simulink model "SF049A_LoaMgr"  (R2013b)
settings: Solver=FixedStepDiscrete  SolverMode=SingleTasking  StartTime=0.0  StopTime=1  FixedStep=0.002  RelTol=1e-3
values from neighbouring files (symbols this model uses):
  CURRMEASLOAMTGTNMASK_CNT_U08 = DataDict.Constant    [SF049A_LoaMgr_DataDict.m]
  IVTRLOAMTGTNMASK_CNT_U08 = DataDict.Constant    [SF049A_LoaMgr_DataDict.m]
  LOAMAXSLEW_ULSPERSEC_F32 = DataDict.Constant    [SF049A_LoaMgr_DataDict.m]
  LoaMgrCurrIvtrMtgtnRate = DataDict.Calibration    [SF049A_LoaMgr_DataDict.m]
  LoaMgrCurrIvtrMtgtnSca = DataDict.Calibration    [SF049A_LoaMgr_DataDict.m]
  LoaMgrCurrIvtrMtgtnScaZeroEna = DataDict.Calibration    [SF049A_LoaMgr_DataDict.m]
  LoaMgrCurrMeasIdptSig0Resp = DataDict.Calibration    [SF049A_LoaMgr_DataDict.m]
  LoaMgrCurrMeasIdptSig1Resp = DataDict.Calibration    [SF049A_LoaMgr_DataDict.m]
  LoaMgrCurrMeasIdptSig2Resp = DataDict.Calibration    [SF049A_LoaMgr_DataDict.m]
  LoaMgrCurrMeasIdptSigFltThd = DataDict.Calibration    [SF049A_LoaMgr_DataDict.m]
  LoaMgrCurrMeasMtgtnRate = DataDict.Calibration    [SF049A_LoaMgr_DataDict.m]
  LoaMgrCurrMeasMtgtnSca = DataDict.Calibration    [SF049A_LoaMgr_DataDict.m]
  LoaMgrCurrMeasMtgtnScaZeroEna = DataDict.Calibration    [SF049A_LoaMgr_DataDict.m]
  LoaMgrFadeOutStRate = DataDict.Calibration    [SF049A_LoaMgr_DataDict.m]
  LoaMgrHwTqIdptSig0NoTqLoaResp = DataDict.Calibration    [SF049A_LoaMgr_DataDict.m]
  LoaMgrHwTqIdptSig1NoTqLoaResp = DataDict.Calibration    [SF049A_LoaMgr_DataDict.m]
  LoaMgrHwTqIdptSig2Resp = DataDict.Calibration    [SF049A_LoaMgr_DataDict.m]
  LoaMgrHwTqIdptSig4Resp = DataDict.Calibration    [SF049A_LoaMgr_DataDict.m]
  LoaMgrHwTqIdptSigFltThd = DataDict.Calibration    [SF049A_LoaMgr_DataDict.m]
  LoaMgrHwTqLoaAvlResp = DataDict.Calibration    [SF049A_LoaMgr_DataDict.m]
  LoaMgrIvtrIdptSig0Resp = DataDict.Calibration    [SF049A_LoaMgr_DataDict.m]
  LoaMgrIvtrIdptSig1Resp = DataDict.Calibration    [SF049A_LoaMgr_DataDict.m]
  LoaMgrIvtrIdptSig2Resp = DataDict.Calibration    [SF049A_LoaMgr_DataDict.m]
  LoaMgrIvtrIdptSigFltThd = DataDict.Calibration    [SF049A_LoaMgr_DataDict.m]
  LoaMgrIvtrMtgtnRate = DataDict.Calibration    [SF049A_LoaMgr_DataDict.m]
  LoaMgrIvtrMtgtnSca = DataDict.Calibration    [SF049A_LoaMgr_DataDict.m]
  LoaMgrIvtrMtgtnScaZeroEna = DataDict.Calibration    [SF049A_LoaMgr_DataDict.m]
  LoaMgrLimdStRate = DataDict.Calibration    [SF049A_LoaMgr_DataDict.m]
  LoaMgrLimdStSca = DataDict.Calibration    [SF049A_LoaMgr_DataDict.m]
  LoaMgrMotAgAvlSnsrlsResp = DataDict.Calibration    [SF049A_LoaMgr_DataDict.m]
  LoaMgrMotAgIdptSig0NoSnsrlsResp = DataDict.Calibration    [SF049A_LoaMgr_DataDict.m]
  LoaMgrMotAgIdptSig1NoSnsrlsResp = DataDict.Calibration    [SF049A_LoaMgr_DataDict.m]
  LoaMgrMotAgIdptSig2Resp = DataDict.Calibration    [SF049A_LoaMgr_DataDict.m]
  LoaMgrMotAgIdptSig3Resp = DataDict.Calibration    [SF049A_LoaMgr_DataDict.m]
  LoaMgrMotAgIdptSigFltThd = DataDict.Calibration    [SF049A_LoaMgr_DataDict.m]
  LoaMgrMotAgMtgtnRate = DataDict.Calibration    [SF049A_LoaMgr_DataDict.m]
  LoaMgrMotAgMtgtnSca = DataDict.Calibration    [SF049A_LoaMgr_DataDict.m]
  LoaMgrMotAgMtgtnScaZeroEna = DataDict.Calibration    [SF049A_LoaMgr_DataDict.m]
  LOASCAONE_ULS_F32 = DataDict.Constant    [SF049A_LoaMgr_DataDict.m]
  LOASCAZERO_ULS_F32 = DataDict.Constant    [SF049A_LoaMgr_DataDict.m]
  LOASTIMDTSHTDWN_CNT_U08 = DataDict.Constant    [SF049A_LoaMgr_DataDict.m]
  LOASTNORM_CNT_U08 = DataDict.Constant    [SF049A_LoaMgr_DataDict.m]
  LOASTSWMTGTN_CNT_U08 = DataDict.Constant    [SF049A_LoaMgr_DataDict.m]
  MAXCURRMEASIDPTSIGALLWD_CNT_U08 = DataDict.Constant    [SF049A_LoaMgr_DataDict.m]
  MAXHWTQIDPTSIGALLWD_CNT_U08 = DataDict.Constant    [SF049A_LoaMgr_DataDict.m]
  MAXIVTRIDPTSIGALLWD_CNT_U08 = DataDict.Constant    [SF049A_LoaMgr_DataDict.m]
  MAXMOTAGMECLIDPTSIGALLWD_CNT_U08 = DataDict.Constant    [SF049A_LoaMgr_DataDict.m]
  NODEBSTEP_CNT_U16 = DataDict.Constant    [SF049A_LoaMgr_DataDict.m]
undefined symbols (not defined in the file or in its folder): LoaSt1, NtcNr1, NtcSts1, SigQlfr1
libraries: simulink x43, NxtrMin x4, NxtrMax x4, NxtrLim x2
(part 7 of 8)

== system SF049A_LoaMgr/LoaMgr/LoaMgrPer1/Request_Responses/MotAgResp/one ==
  MotAgAvlSnsrlsResp : Inport
  MotAgIdptSig1NoResp : Inport  Port=2
  MotAgAvlSnsrls : Inport  Port=3
  one : ActionPort  ActionType=case
  " " : Merge  RequirementInfo="{'linktype_rmi_doors' '0000bab3 (/E-STEER Core/SubSystem Specifications/Application Functions/SF049A Loss of Assist Manager)' '#SF049A_183' 'true' 'REQ:  SF049A_183' '' } %GIDa_4182a502_c274_4352_b30c_44918a836976"
  CopyRight2 : Subsystem  Description=|  mask(Copyright Information){none=on}
      | Copyright info block.                                               
      |                                                                     
      | Place copyright information at the top of every subsystem in design.
      mask prompts: none "No parameters"
      mask help: Place copyright information at the top of every subsystem in design.
      mask Display:
      | NxtrConf = 'Nexteer Confidential';
      | 
      | sys = bdroot; %handle for the current model ("system")
      | first = get_param(sys,'Created');
      | first = first(end-3:end);  %year is last four digits
      | 
      | last = get_param(sys,'LastModifiedDate');
      | if isempty(last)
      |     last = datestr(now,'yyyy');
      | else
      |     last = last(end-3:end);
      | end
      | 
      | if strcmp(first,last)
      |     fprintf('%s -- Copyright %s Nexteer',NxtrConf,first)
      | else
      |     fprintf('%s -- %s%s- %s Nexteer',NxtrConf,char(169),first,last)
      | end
  Ivtr1Inactv_IF : If  RequirementInfo="{'linktype_rmi_doors' '0000bab3 (/E-STEER Core/SubSystem Specifications/Application Functions/SF049A Loss of Assist Manager)' '#SF049A_183' 'true' 'REQ:  SF049A_183' '' } %GIDa_d9c4d673_0ab1_4232_be5c_95383af81f7c"  IfExpression=u1
  cal1 : Subsystem  RequirementInfo="{'linktype_rmi_doors' '0000bab3 (/E-STEER Core/SubSystem Specifications/Application Functions/SF049A Loss of Assist Manager)' '#SF049A_183' 'true' 'REQ:  SF049A_183' '' } %GIDa_64953195_8878_4b1c_98ab_73167e7d198e"  TreatAsAtomicUnit=on
      settings: RTWSystemCode=Inline
  cal2 : Subsystem  RequirementInfo="{'linktype_rmi_doors' '0000bab3 (/E-STEER Core/SubSystem Specifications/Application Functions/SF049A Loss of Assist Manager)' '#SF049A_183' 'true' 'REQ:  SF049A_183' '' } %GIDa_9b0a2cdc_50bc_461c_be5e_30bc8b3ac44b"  TreatAsAtomicUnit=on
      settings: RTWSystemCode=Inline
  MotAgResp : Outport
  wires:
  " "/1 -> MotAgResp/1
  MotAgIdptSig1NoResp/1 -> cal2/1(In1)
  MotAgAvlSnsrlsResp/1 -> cal1/1(In1)
  cal1/1(Out2) -> " "/1
  MotAgAvlSnsrls/1 -> Ivtr1Inactv_IF/1
  cal2/1(Out1) -> " "/2
  Ivtr1Inactv_IF/1 -> cal1/Action
  Ivtr1Inactv_IF/2 -> cal2/Action

== system SF049A_LoaMgr/LoaMgr/LoaMgrPer1/Set_Faults/NTC_Fault1/SetNtcSts ==
  NtcNr : Inport
  NtcStInfo : Inport  Port=2
  NtcSts : Inport  Port=3
  DebStep : Inport  Port=4
  CopyRight2 : Subsystem  Description=|  mask(Copyright Information){none=on}
      | Copyright info block.                                               
      |                                                                     
      | Place copyright information at the top of every subsystem in design.
      mask prompts: none "No parameters"
      mask help: Place copyright information at the top of every subsystem in design.
      mask Display:
      | NxtrConf = 'Nexteer Confidential';
      | 
      | sys = bdroot; %handle for the current model ("system")
      | first = get_param(sys,'Created');
      | first = first(end-3:end);  %year is last four digits
      | 
      | last = get_param(sys,'LastModifiedDate');
      | if isempty(last)
      |     last = datestr(now,'yyyy');
      | else
      |     last = last(end-3:end);
      | end
      | 
      | if strcmp(first,last)
      |     fprintf('%s -- Copyright %s Nexteer',NxtrConf,first)
      | else
      |     fprintf('%s -- %s%s- %s Nexteer',NxtrConf,char(169),first,last)
      | end
  Data Store Write1 : DataStoreWrite  DataStoreName=DebStep
  Data Store Write3 : DataStoreWrite  DataStoreName=Fault1_Status
  Terminator : Terminator
  Terminator1 : Terminator
  wires:
  NtcStInfo/1 -> Terminator1/1
  NtcNr/1 -> Terminator/1
  NtcSts/1 -> Data Store Write3/1
  DebStep/1 -> Data Store Write1/1

== system SF049A_LoaMgr/LoaMgr/LoaMgrPer1/Set_Faults/NTC_Fault2/SetNtcSts ==
  NtcNr : Inport
  NtcStInfo : Inport  Port=2
  NtcSts : Inport  Port=3
  DebStep : Inport  Port=4
  CopyRight2 : Subsystem  Description=|  mask(Copyright Information){none=on}
      | Copyright info block.                                               
      |                                                                     
      | Place copyright information at the top of every subsystem in design.
      mask prompts: none "No parameters"
      mask help: Place copyright information at the top of every subsystem in design.
      mask Display:
      | NxtrConf = 'Nexteer Confidential';
      | 
      | sys = bdroot; %handle for the current model ("system")
      | first = get_param(sys,'Created');
      | first = first(end-3:end);  %year is last four digits
      | 
      | last = get_param(sys,'LastModifiedDate');
      | if isempty(last)
      |     last = datestr(now,'yyyy');
      | else
      |     last = last(end-3:end);
      | end
      | 
      | if strcmp(first,last)
      |     fprintf('%s -- Copyright %s Nexteer',NxtrConf,first)
      | else
      |     fprintf('%s -- %s%s- %s Nexteer',NxtrConf,char(169),first,last)
      | end
  Data Store Write1 : DataStoreWrite  DataStoreName=DebStep
  Data Store Write3 : DataStoreWrite  DataStoreName=Fault2_Status
  Terminator : Terminator
  Terminator1 : Terminator
  wires:
  DebStep/1 -> Data Store Write1/1
  NtcSts/1 -> Data Store Write3/1
  NtcNr/1 -> Terminator/1
  NtcStInfo/1 -> Terminator1/1

== system SF049A_LoaMgr/LoaMgr/LoaMgrPer1/Set_Faults/NTC_Fault3/SetNtcSts ==
  NtcNr : Inport
  NtcStInfo : Inport  Port=2
  NtcSts : Inport  Port=3
  DebStep : Inport  Port=4
  CopyRight2 : Subsystem  Description=|  mask(Copyright Information){none=on}
      | Copyright info block.                                               
      |                                                                     
      | Place copyright information at the top of every subsystem in design.
      mask prompts: none "No parameters"
      mask help: Place copyright information at the top of every subsystem in design.
      mask Display:
      | NxtrConf = 'Nexteer Confidential';
      | 
      | sys = bdroot; %handle for the current model ("system")
      | first = get_param(sys,'Created');
      | first = first(end-3:end);  %year is last four digits
      | 
      | last = get_param(sys,'LastModifiedDate');
      | if isempty(last)
      |     last = datestr(now,'yyyy');
      | else
      |     last = last(end-3:end);
      | end
      | 
      | if strcmp(first,last)
      |     fprintf('%s -- Copyright %s Nexteer',NxtrConf,first)
      | else
      |     fprintf('%s -- %s%s- %s Nexteer',NxtrConf,char(169),first,last)
      | end
  Data Store Write1 : DataStoreWrite  DataStoreName=DebStep
  Data Store Write3 : DataStoreWrite  DataStoreName=Fault3_Status
  Terminator : Terminator
  Terminator1 : Terminator
  wires:
  DebStep/1 -> Data Store Write1/1
  NtcSts/1 -> Data Store Write3/1
  NtcNr/1 -> Terminator/1
  NtcStInfo/1 -> Terminator1/1

== system SF049A_LoaMgr/LoaMgr/LoaMgrPer1/Set_Faults/NTC_Fault4/SetNtcSts ==
  NtcNr : Inport
  NtcStInfo : Inport  Port=2
  NtcSts : Inport  Port=3
  DebStep : Inport  Port=4
  CopyRight2 : Subsystem  Description=|  mask(Copyright Information){none=on}
      | Copyright info block.                                               
      |                                                                     
      | Place copyright information at the top of every subsystem in design.
      mask prompts: none "No parameters"
      mask help: Place copyright information at the top of every subsystem in design.
      mask Display:
      | NxtrConf = 'Nexteer Confidential';
      | 
      | sys = bdroot; %handle for the current model ("system")
      | first = get_param(sys,'Created');
      | first = first(end-3:end);  %year is last four digits
      | 
      | last = get_param(sys,'LastModifiedDate');
      | if isempty(last)
      |     last = datestr(now,'yyyy');
      | else
      |     last = last(end-3:end);
      | end
      | 
      | if strcmp(first,last)
      |     fprintf('%s -- Copyright %s Nexteer',NxtrConf,first)
      | else
      |     fprintf('%s -- %s%s- %s Nexteer',NxtrConf,char(169),first,last)
      | end
  Data Store Write1 : DataStoreWrite  DataStoreName=DebStep
  Data Store Write3 : DataStoreWrite  DataStoreName=Fault4_Status
  Terminator : Terminator
  Terminator1 : Terminator
  wires:
  NtcStInfo/1 -> Terminator1/1
  NtcNr/1 -> Terminator/1
  NtcSts/1 -> Data Store Write3/1
  DebStep/1 -> Data Store Write1/1

== system SF049A_LoaMgr/LoaMgr/LoaMgrPer1/Set_Faults/NTC_Fault5/CopyRight2 ==

== system SF049A_LoaMgr/LoaMgr/LoaMgrPer1/Set_Faults/NTC_Fault6/CopyRight2 ==

== system SF049A_LoaMgr/LoaMgr/LoaMgrPer1/Arbitrate_Responses/CntSwBasdMtgtn/CntMtgtnReq/CopyRight2 ==

== system SF049A_LoaMgr/LoaMgr/LoaMgrPer1/Arbitrate_Responses/CntSwBasdMtgtn/CntMtgtnReq/HwTq_ELSE ==
  In1 : Inport
  Action Port : ActionPort  ActionType=else
  Out1 : Outport
  wires:
  In1/1 -> Out1/1

== system SF049A_LoaMgr/LoaMgr/LoaMgrPer1/Arbitrate_Responses/CntSwBasdMtgtn/CntMtgtnReq/HwTq_THEN ==
  In1 : Inport
  Action Port : ActionPort  ActionType=then
  Out1 : Outport
  wires:
  In1/1 -> Out1/1

== system SF049A_LoaMgr/LoaMgr/LoaMgrPer1/Arbitrate_Responses/CntSwBasdMtgtn/CntMtgtnReq/MotAg_ELSE ==
  In1 : Inport
  Action Port : ActionPort  ActionType=else
  Out1 : Outport
  wires:
  In1/1 -> Out1/1

== system SF049A_LoaMgr/LoaMgr/LoaMgrPer1/Arbitrate_Responses/CntSwBasdMtgtn/CntMtgtnReq/MotAg_THEN ==
  In1 : Inport
  Action Port : ActionPort  ActionType=then
  Out1 : Outport
  wires:
  In1/1 -> Out1/1

== system SF049A_LoaMgr/LoaMgr/LoaMgrPer1/Arbitrate_Responses/CntSwBasdMtgtn/CntMtgtnReq/VltgModReq_ELSE ==
  In1 : Inport
  Action Port : ActionPort  ActionType=else
  Out1 : Outport
  wires:
  In1/1 -> Out1/1

== system SF049A_LoaMgr/LoaMgr/LoaMgrPer1/Arbitrate_Responses/CntSwBasdMtgtn/CntMtgtnReq/VltgModReq_THEN ==
  In1 : Inport
  Action Port : ActionPort  ActionType=then
  Out1 : Outport
  wires:
  In1/1 -> Out1/1

== system SF049A_LoaMgr/LoaMgr/LoaMgrPer1/Arbitrate_Responses/CntSwBasdMtgtn/IllegalCombination/CopyRight2 ==

== system SF049A_LoaMgr/LoaMgr/LoaMgrPer1/Arbitrate_Responses/CntSwBasdMtgtn/OK_to_use/CopyRight2 ==

== system SF049A_LoaMgr/LoaMgr/LoaMgrPer1/Arbitrate_Responses/SelFinalResp/F1/CopyRight2 ==

== system SF049A_LoaMgr/LoaMgr/LoaMgrPer1/Arbitrate_Responses/SelFinalResp/F2/CopyRight2 ==

== system SF049A_LoaMgr/LoaMgr/LoaMgrPer1/Arbitrate_Responses/SelFinalResp/Fade_Out/CopyRight2 ==

== system SF049A_LoaMgr/LoaMgr/LoaMgrPer1/Arbitrate_Responses/SelFinalResp/Fade_Out1/CopyRight2 ==

== system SF049A_LoaMgr/LoaMgr/LoaMgrPer1/Arbitrate_Responses/SelFinalResp/Norm/CopyRight2 ==

== system SF049A_LoaMgr/LoaMgr/LoaMgrPer1/Arbitrate_Responses/SelFinalResp/Reduced/CopyRight2 ==

== system SF049A_LoaMgr/LoaMgr/LoaMgrPer1/Arbitrate_Responses/SelFinalResp/SwBasd_Mtgtn/CopyRight2 ==

== system SF049A_LoaMgr/LoaMgr/LoaMgrPer1/Assign_Scale/SwMtgtn/HwTqTrue/CopyRight2 ==

== system SF049A_LoaMgr/LoaMgr/LoaMgrPer1/Assign_Scale/SwMtgtn/MaskBooleans/CopyRight2 ==

== system SF049A_LoaMgr/LoaMgr/LoaMgrPer1/Assign_Scale/SwMtgtn/MaskBooleans/CurrMeas_ELSE ==
  In1 : Inport
  Action Port : ActionPort  ActionType=else
  Out1 : Outport
  wires:
  In1/1 -> Out1/1

== system SF049A_LoaMgr/LoaMgr/LoaMgrPer1/Assign_Scale/SwMtgtn/MaskBooleans/CurrMeas_THEN ==
  In1 : Inport
  Action Port : ActionPort  ActionType=then
  Out1 : Outport
  wires:
  In1/1 -> Out1/1

== system SF049A_LoaMgr/LoaMgr/LoaMgrPer1/Assign_Scale/SwMtgtn/MaskBooleans/Ivtr_ELSE ==
  In1 : Inport
  Action Port : ActionPort  ActionType=else
  Out1 : Outport
  wires:
  In1/1 -> Out1/1

== system SF049A_LoaMgr/LoaMgr/LoaMgrPer1/Assign_Scale/SwMtgtn/MaskBooleans/Ivtr_THEN ==
  In1 : Inport
  Action Port : ActionPort  ActionType=then
  Out1 : Outport
  wires:
  In1/1 -> Out1/1

== system SF049A_LoaMgr/LoaMgr/LoaMgrPer1/Assign_Scale/SwMtgtn/MotAgTrue/CopyRight2 ==

== system SF049A_LoaMgr/LoaMgr/LoaMgrPer1/Assign_Scale/SwMtgtn/MotAgTrue/PassThru1 ==
  In1 : Inport
  In2 : Inport  Port=2
  Action Port : ActionPort  ActionType=then
  Sca : Outport
  Rate : Outport  Port=2
  wires:
  In1/1 -> Sca/1
  In2/1 -> Rate/1

== system SF049A_LoaMgr/LoaMgr/LoaMgrPer1/Assign_Scale/SwMtgtn/MotAgTrue/PassThru2 ==
  In1 : Inport
  In2 : Inport  Port=2
  Action Port : ActionPort  ActionType=else
  Sca : Outport
  Rate : Outport  Port=2
  wires:
  In1/1 -> Sca/1
  In2/1 -> Rate/1

== system SF049A_LoaMgr/LoaMgr/LoaMgrPer1/Assign_Scale/SwMtgtn/OthersTrue/CopyRight2 ==

== system SF049A_LoaMgr/LoaMgr/LoaMgrPer1/Assign_Scale/SwMtgtn/OthersTrue/CurrIvtr ==
  NewValFlg : Inport  RequirementInfo="{'linktype_rmi_doors' '0000bab3 (/E-STEER Core/SubSystem Specifications/Application Functions/SF049A Loss of Assist Manager)' '#SF049A_107' 'true' 'REQ:  SF049A_107' '' } %GIDa_e92ac1af_0296_4258_8e06_232be688a8c1"
  Action Port : ActionPort  ActionType=case
  Constant1 : Constant  RequirementInfo="{'linktype_rmi_doors' '0000bab3 (/E-STEER Core/SubSystem Specifications/Application Functions/SF049A Loss of Assist Manager)' '#SF049A_104' 'true' 'REQ:  SF049A_104' '' ; 'linktype_rmi_doors' '0000bab3 (/E-STEER Core/SubSystem Specifications/Application Functions/SF049A Loss of Assist Manager)' '#SF049A_107' 'true' 'REQ:  SF049A_107' '' ; 'linktype_rmi_doors' '0000bab3 (/E-STEER Core/SubSystem Specifications/Application Functions/SF049A Loss of Assist Manager)' '#SF049A_108' 'true' 'REQ:  SF049A_108' '' } %GIDa_0a7f0acf_b35d_434a_8dc6_ba391d17eb63"  Value=LoaMgrCurrIvtrMtgtnRate
  Constant3 : Constant  RequirementInfo="{'linktype_rmi_doors' '0000bab3 (/E-STEER Core/SubSystem Specifications/Application Functions/SF049A Loss of Assist Manager)' '#SF049A_107' 'true' 'REQ:  SF049A_107' '' } %GIDa_4edd071c_4397_4e3b_a07a_efc9ca10b177"  Value=LOASCAZERO_ULS_F32
  Constant4 : Constant  RequirementInfo="{'linktype_rmi_doors' '0000bab3 (/E-STEER Core/SubSystem Specifications/Application Functions/SF049A Loss of Assist Manager)' '#SF049A_107' 'true' 'REQ:  SF049A_107' '' } %GIDa_e2b66e7c_9ee8_43b1_b96c_e0e22fd25a1e"  Value=LOAMAXSLEW_ULSPERSEC_F32
  Constant5 : Constant  RequirementInfo="{'linktype_rmi_doors' '0000bab3 (/E-STEER Core/SubSystem Specifications/Application Functions/SF049A Loss of Assist Manager)' '#SF049A_105' 'true' 'REQ:  SF049A_105' '' ; 'linktype_rmi_doors' '0000bab3 (/E-STEER Core/SubSystem Specifications/Application Functions/SF049A Loss of Assist Manager)' '#SF049A_107' 'true' 'REQ:  SF049A_107' '' ; 'linktype_rmi_doors' '0000bab3 (/E-STEER Core/SubSystem Specifications/Application Functions/SF049A Loss of Assist Manager)' '#SF049A_108' 'true' 'REQ:  SF049A_108' '' } %GIDa_066a9c65_452a_4614_b67a_f19d7754eaec"  Value=LoaMgrCurrIvtrMtgtnScaZeroEna
  Constant6 : Constant  RequirementInfo="{'linktype_rmi_doors' '0000bab3 (/E-STEER Core/SubSystem Specifications/Application Functions/SF049A Loss of Assist Manager)' '#SF049A_104' 'true' 'REQ:  SF049A_104' '' ; 'linktype_rmi_doors' '0000bab3 (/E-STEER Core/SubSystem Specifications/Application Functions/SF049A Loss of Assist Manager)' '#SF049A_107' 'true' 'REQ:  SF049A_107' '' ; 'linktype_rmi_doors' '0000bab3 (/E-STEER Core/SubSystem Specifications/Application Functions/SF049A Loss of Assist Manager)' '#SF049A_108' 'true' 'REQ:  SF049A_108' '' } %GIDa_98c21134_9a78_4cbf_aa34_e5c0f5405f23"  Value=LoaMgrCurrIvtrMtgtnSca
  CopyRight2 : Subsystem  Description=|  mask(Copyright Information){none=on}
      | Copyright info block.                                               
      |                                                                     
      | Place copyright information at the top of every subsystem in design.
      mask prompts: none "No parameters"
      mask help: Place copyright information at the top of every subsystem in design.
      mask Display:
      | NxtrConf = 'Nexteer Confidential';
      | 
      | sys = bdroot; %handle for the current model ("system")
      | first = get_param(sys,'Created');
      | first = first(end-3:end);  %year is last four digits
      | 
      | last = get_param(sys,'LastModifiedDate');
      | if isempty(last)
      |     last = datestr(now,'yyyy');
      | else
      |     last = last(end-3:end);
      | end
      | 
      | if strcmp(first,last)
      |     fprintf('%s -- Copyright %s Nexteer',NxtrConf,first)
      | else
      |     fprintf('%s -- %s%s- %s Nexteer',NxtrConf,char(169),first,last)
      | end
  If : If  RequirementInfo="{'linktype_rmi_doors' '0000bab3 (/E-STEER Core/SubSystem Specifications/Application Functions/SF049A Loss of Assist Manager)' '#SF049A_107' 'true' 'REQ:  SF049A_107' '' ; 'linktype_rmi_doors' '0000bab3 (/E-STEER Core/SubSystem Specifications/Application Functions/SF049A Loss of Assist Manager)' '#SF049A_108' 'true' 'REQ:  SF049A_108' '' } %GIDa_d8db09ca_83f4_4349_b4d4_b98e816c5376"  NumInputs=2  IfExpression=u1 & u2
  PassThru1 : Subsystem  RequirementInfo="{'linktype_rmi_doors' '0000bab3 (/E-STEER Core/SubSystem Specifications/Application Functions/SF049A Loss of Assist Manager)' '#SF049A_107' 'true' 'REQ:  SF049A_107' '' } %GIDa_f3e1234b_6b2b_42dd_80fa_22b05716026b"  TreatAsAtomicUnit=on
  PassThru2 : Subsystem  RequirementInfo="{'linktype_rmi_doors' '0000bab3 (/E-STEER Core/SubSystem Specifications/Application Functions/SF049A Loss of Assist Manager)' '#SF049A_107' 'true' 'REQ:  SF049A_107' '' ; 'linktype_rmi_doors' '0000bab3 (/E-STEER Core/SubSystem Specifications/Application Functions/SF049A Loss of Assist Manager)' '#SF049A_108' 'true' 'REQ:  SF049A_108' '' } %GIDa_ed7fbb5a_efd5_4599_a480_5dcaca990a0b"  TreatAsAtomicUnit=on
  RateMerge : Merge  RequirementInfo="{'linktype_rmi_doors' '0000bab3 (/E-STEER Core/SubSystem Specifications/Application Functions/SF049A Loss of Assist Manager)' '#SF049A_107' 'true' 'REQ:  SF049A_107' '' ; 'linktype_rmi_doors' '0000bab3 (/E-STEER Core/SubSystem Specifications/Application Functions/SF049A Loss of Assist Manager)' '#SF049A_108' 'true' 'REQ:  SF049A_108' '' } %GIDa_9a5d542a_8c6b_48df_adb4_ce3edcbd33ae"
  ScaMerge : Merge  RequirementInfo="{'linktype_rmi_doors' '0000bab3 (/E-STEER Core/SubSystem Specifications/Application Functions/SF049A Loss of Assist Manager)' '#SF049A_107' 'true' 'REQ:  SF049A_107' '' ; 'linktype_rmi_doors' '0000bab3 (/E-STEER Core/SubSystem Specifications/Application Functions/SF049A Loss of Assist Manager)' '#SF049A_108' 'true' 'REQ:  SF049A_108' '' } %GIDa_cd99e34c_49c0_43cc_a644_ad48e1f7d865"
  Sca : Outport  RequirementInfo="{'linktype_rmi_doors' '0000bab3 (/E-STEER Core/SubSystem Specifications/Application Functions/SF049A Loss of Assist Manager)' '#SF049A_107' 'true' 'REQ:  SF049A_107' '' ; 'linktype_rmi_doors' '0000bab3 (/E-STEER Core/SubSystem Specifications/Application Functions/SF049A Loss of Assist Manager)' '#SF049A_108' 'true' 'REQ:  SF049A_108' '' } %GIDa_bf14eed3_0593_4136_9c2c_10e7a1309ce3"
  Rate : Outport  RequirementInfo="{'linktype_rmi_doors' '0000bab3 (/E-STEER Core/SubSystem Specifications/Application Functions/SF049A Loss of Assist Manager)' '#SF049A_107' 'true' 'REQ:  SF049A_107' '' ; 'linktype_rmi_doors' '0000bab3 (/E-STEER Core/SubSystem Specifications/Application Functions/SF049A Loss of Assist Manager)' '#SF049A_108' 'true' 'REQ:  SF049A_108' '' } %GIDa_8b01cc54_9dbd_4d50_adf4_3a0f71775263"  Port=2
  wires:
  ScaMerge/1 -> Sca/1
  RateMerge/1 -> Rate/1
  NewValFlg/1 -> If/1
  Constant5/1 -> If/2
  Constant3/1 -> PassThru1/1(In1)
  Constant4/1 -> PassThru1/2(In2)
  Constant6/1 -> PassThru2/1(In1)
  Constant1/1 -> PassThru2/2(In2)
  If/1 -> PassThru1/Action
  If/2 -> PassThru2/Action
  PassThru1/1(Sca) -> ScaMerge/1
  PassThru1/2(Rate) -> RateMerge/1
  PassThru2/1(Sca) -> ScaMerge/2
  PassThru2/2(Rate) -> RateMerge/2

== system SF049A_LoaMgr/LoaMgr/LoaMgrPer1/Assign_Scale/SwMtgtn/OthersTrue/CurrOnly ==
  note: IF NewValFlag and Cal are both True THEN
      |      Target scale factor is Zero
      |      Slew rate is instantaneous
      | ELSE
      |      Target scale factor is a cal value
      |      Slew rate is a cal value
      | ENDIF
  note: We could only reach this routine when the combination of s/w-based mitigations changed, making the NewValFlag true.
      | When the flag is true the user may want to drop scale factor instantly to zero and then ramp back up to a target.
  note: If we enter this block on the next loop, the NewValFlag will be FALSE because of the current loop.
      | The user's calibrated scale factor and slew rate will be used.  This means that the slew rate is
      | applied whether the system is slewing down from ONE or up from ZERO.
  NewValFlg : Inport  RequirementInfo="{'linktype_rmi_doors' '0000bab3 (/E-STEER Core/SubSystem Specifications/Application Functions/SF049A Loss of Assist Manager)' '#SF049A_107' 'true' 'REQ:  SF049A_107' '' } %GIDa_362b74b3_57a1_4d55_99eb_b4a3317b4ca7"
  Action Port : ActionPort  ActionType=case
  Constant1 : Constant  RequirementInfo="{'linktype_rmi_doors' '0000bab3 (/E-STEER Core/SubSystem Specifications/Application Functions/SF049A Loss of Assist Manager)' '#SF049A_104' 'true' 'REQ:  SF049A_104' '' ; 'linktype_rmi_doors' '0000bab3 (/E-STEER Core/SubSystem Specifications/Application Functions/SF049A Loss of Assist Manager)' '#SF049A_107' 'true' 'REQ:  SF049A_107' '' ; 'linktype_rmi_doors' '0000bab3 (/E-STEER Core/SubSystem Specifications/Application Functions/SF049A Loss of Assist Manager)' '#SF049A_108' 'true' 'REQ:  SF049A_108' '' } %GIDa_9c03c4aa_189f_4633_8df5_340fd1279f4e"  Value=LoaMgrCurrMeasMtgtnRate
  Constant3 : Constant  RequirementInfo="{'linktype_rmi_doors' '0000bab3 (/E-STEER Core/SubSystem Specifications/Application Functions/SF049A Loss of Assist Manager)' '#SF049A_107' 'true' 'REQ:  SF049A_107' '' } %GIDa_b3be7be0_cd2a_4a95_8fea_ee44dd6244d6"  Value=LOASCAZERO_ULS_F32
  Constant4 : Constant  RequirementInfo="{'linktype_rmi_doors' '0000bab3 (/E-STEER Core/SubSystem Specifications/Application Functions/SF049A Loss of Assist Manager)' '#SF049A_107' 'true' 'REQ:  SF049A_107' '' } %GIDa_e0fded85_7cf9_4e33_802e_54b379993a78"  Value=LOAMAXSLEW_ULSPERSEC_F32
  Constant5 : Constant  RequirementInfo="{'linktype_rmi_doors' '0000bab3 (/E-STEER Core/SubSystem Specifications/Application Functions/SF049A Loss of Assist Manager)' '#SF049A_105' 'true' 'REQ:  SF049A_105' '' ; 'linktype_rmi_doors' '0000bab3 (/E-STEER Core/SubSystem Specifications/Application Functions/SF049A Loss of Assist Manager)' '#SF049A_107' 'true' 'REQ:  SF049A_107' '' ; 'linktype_rmi_doors' '0000bab3 (/E-STEER Core/SubSystem Specifications/Application Functions/SF049A Loss of Assist Manager)' '#SF049A_108' 'true' 'REQ:  SF049A_108' '' } %GIDa_7cf2ac86_d907_4ba2_9fb2_6c85d9245d24"  Value=LoaMgrCurrMeasMtgtnScaZeroEna
  Constant6 : Constant  RequirementInfo="{'linktype_rmi_doors' '0000bab3 (/E-STEER Core/SubSystem Specifications/Application Functions/SF049A Loss of Assist Manager)' '#SF049A_104' 'true' 'REQ:  SF049A_104' '' ; 'linktype_rmi_doors' '0000bab3 (/E-STEER Core/SubSystem Specifications/Application Functions/SF049A Loss of Assist Manager)' '#SF049A_107' 'true' 'REQ:  SF049A_107' '' ; 'linktype_rmi_doors' '0000bab3 (/E-STEER Core/SubSystem Specifications/Application Functions/SF049A Loss of Assist Manager)' '#SF049A_108' 'true' 'REQ:  SF049A_108' '' } %GIDa_8c90c9f5_5175_4ccd_b857_af290ef7e8ee"  Value=LoaMgrCurrMeasMtgtnSca
  CopyRight2 : Subsystem  Description=|  mask(Copyright Information){none=on}
      | Copyright info block.                                               
      |                                                                     
      | Place copyright information at the top of every subsystem in design.
      mask prompts: none "No parameters"
      mask help: Place copyright information at the top of every subsystem in design.
      mask Display:
      | NxtrConf = 'Nexteer Confidential';
      | 
      | sys = bdroot; %handle for the current model ("system")
      | first = get_param(sys,'Created');
      | first = first(end-3:end);  %year is last four digits
      | 
      | last = get_param(sys,'LastModifiedDate');
      | if isempty(last)
      |     last = datestr(now,'yyyy');
      | else
      |     last = last(end-3:end);
      | end
      | 
      | if strcmp(first,last)
      |     fprintf('%s -- Copyright %s Nexteer',NxtrConf,first)
      | else
      |     fprintf('%s -- %s%s- %s Nexteer',NxtrConf,char(169),first,last)
      | end
  If : If  RequirementInfo="{'linktype_rmi_doors' '0000bab3 (/E-STEER Core/SubSystem Specifications/Application Functions/SF049A Loss of Assist Manager)' '#SF049A_107' 'true' 'REQ:  SF049A_107' '' ; 'linktype_rmi_doors' '0000bab3 (/E-STEER Core/SubSystem Specifications/Application Functions/SF049A Loss of Assist Manager)' '#SF049A_108' 'true' 'REQ:  SF049A_108' '' } %GIDa_a39bedb6_fe38_4bf4_a245_c986718d99d2"  NumInputs=2  IfExpression=u1 & u2
  PassThru1 : Subsystem  RequirementInfo="{'linktype_rmi_doors' '0000bab3 (/E-STEER Core/SubSystem Specifications/Application Functions/SF049A Loss of Assist Manager)' '#SF049A_107' 'true' 'REQ:  SF049A_107' '' } %GIDa_92527005_828e_48ae_b2de_ff17012267b2"  TreatAsAtomicUnit=on
  PassThru2 : Subsystem  RequirementInfo="{'linktype_rmi_doors' '0000bab3 (/E-STEER Core/SubSystem Specifications/Application Functions/SF049A Loss of Assist Manager)' '#SF049A_107' 'true' 'REQ:  SF049A_107' '' ; 'linktype_rmi_doors' '0000bab3 (/E-STEER Core/SubSystem Specifications/Application Functions/SF049A Loss of Assist Manager)' '#SF049A_108' 'true' 'REQ:  SF049A_108' '' } %GIDa_54595c34_425d_4567_8e06_8e699962e312"  TreatAsAtomicUnit=on
  RateMerge : Merge  RequirementInfo="{'linktype_rmi_doors' '0000bab3 (/E-STEER Core/SubSystem Specifications/Application Functions/SF049A Loss of Assist Manager)' '#SF049A_107' 'true' 'REQ:  SF049A_107' '' ; 'linktype_rmi_doors' '0000bab3 (/E-STEER Core/SubSystem Specifications/Application Functions/SF049A Loss of Assist Manager)' '#SF049A_108' 'true' 'REQ:  SF049A_108' '' } %GIDa_a7363e1c_672f_4d3a_9088_8b3b02834d62"
  ScaMerge : Merge  RequirementInfo="{'linktype_rmi_doors' '0000bab3 (/E-STEER Core/SubSystem Specifications/Application Functions/SF049A Loss of Assist Manager)' '#SF049A_107' 'true' 'REQ:  SF049A_107' '' ; 'linktype_rmi_doors' '0000bab3 (/E-STEER Core/SubSystem Specifications/Application Functions/SF049A Loss of Assist Manager)' '#SF049A_108' 'true' 'REQ:  SF049A_108' '' } %GIDa_6e0c1319_377a_4b5a_ab50_2ecbc15fc808"
  Sca : Outport  RequirementInfo="{'linktype_rmi_doors' '0000bab3 (/E-STEER Core/SubSystem Specifications/Application Functions/SF049A Loss of Assist Manager)' '#SF049A_107' 'true' 'REQ:  SF049A_107' '' ; 'linktype_rmi_doors' '0000bab3 (/E-STEER Core/SubSystem Specifications/Application Functions/SF049A Loss of Assist Manager)' '#SF049A_108' 'true' 'REQ:  SF049A_108' '' } %GIDa_8759d6d4_2d87_45d5_a984_bf18b48722bc"
  Rate : Outport  RequirementInfo="{'linktype_rmi_doors' '0000bab3 (/E-STEER Core/SubSystem Specifications/Application Functions/SF049A Loss of Assist Manager)' '#SF049A_107' 'true' 'REQ:  SF049A_107' '' ; 'linktype_rmi_doors' '0000bab3 (/E-STEER Core/SubSystem Specifications/Application Functions/SF049A Loss of Assist Manager)' '#SF049A_108' 'true' 'REQ:  SF049A_108' '' } %GIDa_f422c6e4_ce4b_48d7_8bf1_a9ed3de5e714"  Port=2
  wires:
  ScaMerge/1 -> Sca/1
  RateMerge/1 -> Rate/1
  NewValFlg/1 -> If/1
  Constant5/1 -> If/2
  Constant3/1 -> PassThru1/1(In1)
  Constant4/1 -> PassThru1/2(In2)
  Constant6/1 -> PassThru2/1(In1)
  Constant1/1 -> PassThru2/2(In2)
  If/1 -> PassThru1/Action
  If/2 -> PassThru2/Action
  PassThru1/1(Sca) -> ScaMerge/1
  PassThru1/2(Rate) -> RateMerge/1
  PassThru2/1(Sca) -> ScaMerge/2
  PassThru2/2(Rate) -> RateMerge/2

== system SF049A_LoaMgr/LoaMgr/LoaMgrPer1/Assign_Scale/SwMtgtn/OthersTrue/Invalid_Number ==
  note: Should not have entered this block at all.
  Action Port : ActionPort  ActionType=default
  Constant1 : Constant  Value=LOAMAXSLEW_ULSPERSEC_F32
  Constant6 : Constant  Value=LOASCAZERO_ULS_F32
  CopyRight2 : Subsystem  Description=|  mask(Copyright Information){none=on}
      | Copyright info block.                                               
      |                                                                     
      | Place copyright information at the top of every subsystem in design.
      mask prompts: none "No parameters"
      mask help: Place copyright information at the top of every subsystem in design.
      mask Display:
      | NxtrConf = 'Nexteer Confidential';
      | 
      | sys = bdroot; %handle for the current model ("system")
      | first = get_param(sys,'Created');
      | first = first(end-3:end);  %year is last four digits
      | 
      | last = get_param(sys,'LastModifiedDate');
      | if isempty(last)
      |     last = datestr(now,'yyyy');
      | else
      |     last = last(end-3:end);
      | end
      | 
      | if strcmp(first,last)
      |     fprintf('%s -- Copyright %s Nexteer',NxtrConf,first)
      | else
      |     fprintf('%s -- %s%s- %s Nexteer',NxtrConf,char(169),first,last)
      | end
  Sca : Outport
  Rate : Outport  Port=2
  wires:
  Constant6/1 -> Sca/1
  Constant1/1 -> Rate/1

== system SF049A_LoaMgr/LoaMgr/LoaMgrPer1/Assign_Scale/SwMtgtn/OthersTrue/IvtrOnly ==
  NewValFlg : Inport  RequirementInfo="{'linktype_rmi_doors' '0000bab3 (/E-STEER Core/SubSystem Specifications/Application Functions/SF049A Loss of Assist Manager)' '#SF049A_107' 'true' 'REQ:  SF049A_107' '' } %GIDa_bebc64cf_067c_4c6e_a2dd_fbd9ead90333"
  Action Port : ActionPort  ActionType=case
  Constant1 : Constant  RequirementInfo="{'linktype_rmi_doors' '0000bab3 (/E-STEER Core/SubSystem Specifications/Application Functions/SF049A Loss of Assist Manager)' '#SF049A_104' 'true' 'REQ:  SF049A_104' '' ; 'linktype_rmi_doors' '0000bab3 (/E-STEER Core/SubSystem Specifications/Application Functions/SF049A Loss of Assist Manager)' '#SF049A_107' 'true' 'REQ:  SF049A_107' '' ; 'linktype_rmi_doors' '0000bab3 (/E-STEER Core/SubSystem Specifications/Application Functions/SF049A Loss of Assist Manager)' '#SF049A_108' 'true' 'REQ:  SF049A_108' '' } %GIDa_9fe335c9_de39_4c21_b500_a6017497dcf4"  Value=LoaMgrIvtrMtgtnRate
  Constant3 : Constant  RequirementInfo="{'linktype_rmi_doors' '0000bab3 (/E-STEER Core/SubSystem Specifications/Application Functions/SF049A Loss of Assist Manager)' '#SF049A_107' 'true' 'REQ:  SF049A_107' '' } %GIDa_809cc0d0_77cd_4171_a53e_5321a3476069"  Value=LOASCAZERO_ULS_F32
  Constant4 : Constant  RequirementInfo="{'linktype_rmi_doors' '0000bab3 (/E-STEER Core/SubSystem Specifications/Application Functions/SF049A Loss of Assist Manager)' '#SF049A_107' 'true' 'REQ:  SF049A_107' '' } %GIDa_c5d1acda_fa0b_4a21_9154_b30a99ceff6f"  Value=LOAMAXSLEW_ULSPERSEC_F32
  Constant5 : Constant  RequirementInfo="{'linktype_rmi_doors' '0000bab3 (/E-STEER Core/SubSystem Specifications/Application Functions/SF049A Loss of Assist Manager)' '#SF049A_105' 'true' 'REQ:  SF049A_105' '' ; 'linktype_rmi_doors' '0000bab3 (/E-STEER Core/SubSystem Specifications/Application Functions/SF049A Loss of Assist Manager)' '#SF049A_107' 'true' 'REQ:  SF049A_107' '' ; 'linktype_rmi_doors' '0000bab3 (/E-STEER Core/SubSystem Specifications/Application Functions/SF049A Loss of Assist Manager)' '#SF049A_108' 'true' 'REQ:  SF049A_108' '' } %GIDa_fb19a774_08ad_4bce_b53c_121862df767a"  Value=LoaMgrIvtrMtgtnScaZeroEna
  Constant6 : Constant  RequirementInfo="{'linktype_rmi_doors' '0000bab3 (/E-STEER Core/SubSystem Specifications/Application Functions/SF049A Loss of Assist Manager)' '#SF049A_104' 'true' 'REQ:  SF049A_104' '' ; 'linktype_rmi_doors' '0000bab3 (/E-STEER Core/SubSystem Specifications/Application Functions/SF049A Loss of Assist Manager)' '#SF049A_107' 'true' 'REQ:  SF049A_107' '' ; 'linktype_rmi_doors' '0000bab3 (/E-STEER Core/SubSystem Specifications/Application Functions/SF049A Loss of Assist Manager)' '#SF049A_108' 'true' 'REQ:  SF049A_108' '' } %GIDa_270fb049_7b6f_4d8d_9f84_100ba23ad415"  Value=LoaMgrIvtrMtgtnSca
  CopyRight2 : Subsystem  Description=|  mask(Copyright Information){none=on}
      | Copyright info block.                                               
      |                                                                     
      | Place copyright information at the top of every subsystem in design.
      mask prompts: none "No parameters"
      mask help: Place copyright information at the top of every subsystem in design.
      mask Display:
      | NxtrConf = 'Nexteer Confidential';
      | 
      | sys = bdroot; %handle for the current model ("system")
      | first = get_param(sys,'Created');
      | first = first(end-3:end);  %year is last four digits
      | 
      | last = get_param(sys,'LastModifiedDate');
      | if isempty(last)
      |     last = datestr(now,'yyyy');
      | else
      |     last = last(end-3:end);
      | end
      | 
      | if strcmp(first,last)
      |     fprintf('%s -- Copyright %s Nexteer',NxtrConf,first)
      | else
      |     fprintf('%s -- %s%s- %s Nexteer',NxtrConf,char(169),first,last)
      | end
  If : If  RequirementInfo="{'linktype_rmi_doors' '0000bab3 (/E-STEER Core/SubSystem Specifications/Application Functions/SF049A Loss of Assist Manager)' '#SF049A_107' 'true' 'REQ:  SF049A_107' '' ; 'linktype_rmi_doors' '0000bab3 (/E-STEER Core/SubSystem Specifications/Application Functions/SF049A Loss of Assist Manager)' '#SF049A_108' 'true' 'REQ:  SF049A_108' '' } %GIDa_2a0d9a1f_07b4_4588_9fc0_fde88872e17e"  NumInputs=2  IfExpression=u1 & u2
  PassThru1 : Subsystem  RequirementInfo="{'linktype_rmi_doors' '0000bab3 (/E-STEER Core/SubSystem Specifications/Application Functions/SF049A Loss of Assist Manager)' '#SF049A_107' 'true' 'REQ:  SF049A_107' '' } %GIDa_70d83f71_c0e6_42ab_9006_8bd8558d35d6"  TreatAsAtomicUnit=on
  PassThru2 : Subsystem  RequirementInfo="{'linktype_rmi_doors' '0000bab3 (/E-STEER Core/SubSystem Specifications/Application Functions/SF049A Loss of Assist Manager)' '#SF049A_107' 'true' 'REQ:  SF049A_107' '' ; 'linktype_rmi_doors' '0000bab3 (/E-STEER Core/SubSystem Specifications/Application Functions/SF049A Loss of Assist Manager)' '#SF049A_108' 'true' 'REQ:  SF049A_108' '' } %GIDa_52d3ce74_bbf1_442e_8a2f_a850c2aa6c21"  TreatAsAtomicUnit=on
  RateMerge : Merge  RequirementInfo="{'linktype_rmi_doors' '0000bab3 (/E-STEER Core/SubSystem Specifications/Application Functions/SF049A Loss of Assist Manager)' '#SF049A_107' 'true' 'REQ:  SF049A_107' '' ; 'linktype_rmi_doors' '0000bab3 (/E-STEER Core/SubSystem Specifications/Application Functions/SF049A Loss of Assist Manager)' '#SF049A_108' 'true' 'REQ:  SF049A_108' '' } %GIDa_70cfab92_36a1_411f_a2d2_31a72af66c09"
  ScaMerge : Merge  RequirementInfo="{'linktype_rmi_doors' '0000bab3 (/E-STEER Core/SubSystem Specifications/Application Functions/SF049A Loss of Assist Manager)' '#SF049A_107' 'true' 'REQ:  SF049A_107' '' ; 'linktype_rmi_doors' '0000bab3 (/E-STEER Core/SubSystem Specifications/Application Functions/SF049A Loss of Assist Manager)' '#SF049A_108' 'true' 'REQ:  SF049A_108' '' } %GIDa_2f50947f_681a_42f4_af68_407099648f00"
  Sca : Outport  RequirementInfo="{'linktype_rmi_doors' '0000bab3 (/E-STEER Core/SubSystem Specifications/Application Functions/SF049A Loss of Assist Manager)' '#SF049A_107' 'true' 'REQ:  SF049A_107' '' ; 'linktype_rmi_doors' '0000bab3 (/E-STEER Core/SubSystem Specifications/Application Functions/SF049A Loss of Assist Manager)' '#SF049A_108' 'true' 'REQ:  SF049A_108' '' } %GIDa_01054ef6_b634_40c1_872a_86938a20e530"
  Rate : Outport  RequirementInfo="{'linktype_rmi_doors' '0000bab3 (/E-STEER Core/SubSystem Specifications/Application Functions/SF049A Loss of Assist Manager)' '#SF049A_107' 'true' 'REQ:  SF049A_107' '' ; 'linktype_rmi_doors' '0000bab3 (/E-STEER Core/SubSystem Specifications/Application Functions/SF049A Loss of Assist Manager)' '#SF049A_108' 'true' 'REQ:  SF049A_108' '' } %GIDa_c20f4c12_0821_4cc7_8beb_831290c3148f"  Port=2
  wires:
  ScaMerge/1 -> Sca/1
  RateMerge/1 -> Rate/1
  NewValFlg/1 -> If/1
  Constant5/1 -> If/2
  Constant3/1 -> PassThru1/1(In1)
  Constant4/1 -> PassThru1/2(In2)
  Constant6/1 -> PassThru2/1(In1)
  Constant1/1 -> PassThru2/2(In2)
  If/1 -> PassThru1/Action
  If/2 -> PassThru2/Action
  PassThru1/1(Sca) -> ScaMerge/1
  PassThru1/2(Rate) -> RateMerge/1
  PassThru2/1(Sca) -> ScaMerge/2
  PassThru2/2(Rate) -> RateMerge/2

== system SF049A_LoaMgr/LoaMgr/LoaMgrPer1/Request_Responses/CurrMeasResp/Two/CopyRight2 ==

== system SF049A_LoaMgr/LoaMgr/LoaMgrPer1/Request_Responses/CurrMeasResp/Zero_or_Invalid/CopyRight2 ==

== system SF049A_LoaMgr/LoaMgr/LoaMgrPer1/Request_Responses/CurrMeasResp/one/CopyRight2 ==

== system SF049A_LoaMgr/LoaMgr/LoaMgrPer1/Request_Responses/HwTqResp/Four/CopyRight2 ==

== system SF049A_LoaMgr/LoaMgr/LoaMgrPer1/Request_Responses/HwTqResp/Two/CopyRight2 ==

== system SF049A_LoaMgr/LoaMgr/LoaMgrPer1/Request_Responses/HwTqResp/Zero_or_Invalid/CopyRight2 ==

== system SF049A_LoaMgr/LoaMgr/LoaMgrPer1/Request_Responses/HwTqResp/Zero_or_Invalid/cal1 ==
  In1 : Inport
  Action Port : ActionPort  ActionType=then
  CopyRight2 : Subsystem  Description=|  mask(Copyright Information){none=on}
      | Copyright info block.                                               
      |                                                                     
      | Place copyright information at the top of every subsystem in design.
      mask prompts: none "No parameters"
      mask help: Place copyright information at the top of every subsystem in design.
      mask Display:
      | NxtrConf = 'Nexteer Confidential';
      | 
      | sys = bdroot; %handle for the current model ("system")
      | first = get_param(sys,'Created');
      | first = first(end-3:end);  %year is last four digits
      | 
      | last = get_param(sys,'LastModifiedDate');
      | if isempty(last)
      |     last = datestr(now,'yyyy');
      | else
      |     last = last(end-3:end);
      | end
      | 
      | if strcmp(first,last)
      |     fprintf('%s -- Copyright %s Nexteer',NxtrConf,first)
      | else
      |     fprintf('%s -- %s%s- %s Nexteer',NxtrConf,char(169),first,last)
      | end
  Out2 : Outport
  wires:
  In1/1 -> Out2/1

== system SF049A_LoaMgr/LoaMgr/LoaMgrPer1/Request_Responses/HwTqResp/Zero_or_Invalid/cal2 ==
  In1 : Inport
  Action Port : ActionPort  ActionType=else
  CopyRight2 : Subsystem  Description=|  mask(Copyright Information){none=on}
      | Copyright info block.                                               
      |                                                                     
      | Place copyright information at the top of every subsystem in design.
      mask prompts: none "No parameters"
      mask help: Place copyright information at the top of every subsystem in design.
      mask Display:
      | NxtrConf = 'Nexteer Confidential';
      | 
      | sys = bdroot; %handle for the current model ("system")
      | first = get_param(sys,'Created');
      | first = first(end-3:end);  %year is last four digits
      | 
      | last = get_param(sys,'LastModifiedDate');
      | if isempty(last)
      |     last = datestr(now,'yyyy');
      | else
      |     last = last(end-3:end);
      | end
      | 
      | if strcmp(first,last)
      |     fprintf('%s -- Copyright %s Nexteer',NxtrConf,first)
      | else
      |     fprintf('%s -- %s%s- %s Nexteer',NxtrConf,char(169),first,last)
      | end
  Out1 : Outport
  wires:
  In1/1 -> Out1/1

== system SF049A_LoaMgr/LoaMgr/LoaMgrPer1/Request_Responses/HwTqResp/one/CopyRight2 ==

== system SF049A_LoaMgr/LoaMgr/LoaMgrPer1/Request_Responses/HwTqResp/one/cal1 ==
  In1 : Inport
  Action Port : ActionPort  ActionType=then
  CopyRight2 : Subsystem  Description=|  mask(Copyright Information){none=on}
      | Copyright info block.                                               
      |                                                                     
      | Place copyright information at the top of every subsystem in design.
      mask prompts: none "No parameters"
      mask help: Place copyright information at the top of every subsystem in design.
      mask Display:
      | NxtrConf = 'Nexteer Confidential';
      | 
      | sys = bdroot; %handle for the current model ("system")
      | first = get_param(sys,'Created');
      | first = first(end-3:end);  %year is last four digits
      | 
      | last = get_param(sys,'LastModifiedDate');
      | if isempty(last)
      |     last = datestr(now,'yyyy');
      | else
      |     last = last(end-3:end);
      | end
      | 
      | if strcmp(first,last)
      |     fprintf('%s -- Copyright %s Nexteer',NxtrConf,first)
      | else
      |     fprintf('%s -- %s%s- %s Nexteer',NxtrConf,char(169),first,last)
      | end
  Out2 : Outport
  wires:
  In1/1 -> Out2/1

== system SF049A_LoaMgr/LoaMgr/LoaMgrPer1/Request_Responses/HwTqResp/one/cal2 ==
  In1 : Inport
  Action Port : ActionPort  ActionType=else
  CopyRight2 : Subsystem  Description=|  mask(Copyright Information){none=on}
      | Copyright info block.                                               
      |                                                                     
      | Place copyright information at the top of every subsystem in design.
      mask prompts: none "No parameters"
      mask help: Place copyright information at the top of every subsystem in design.
      mask Display:
      | NxtrConf = 'Nexteer Confidential';
      | 
      | sys = bdroot; %handle for the current model ("system")
      | first = get_param(sys,'Created');
      | first = first(end-3:end);  %year is last four digits
      | 
      | last = get_param(sys,'LastModifiedDate');
      | if isempty(last)
      |     last = datestr(now,'yyyy');
      | else
      |     last = last(end-3:end);
      | end
      | 
      | if strcmp(first,last)
      |     fprintf('%s -- Copyright %s Nexteer',NxtrConf,first)
      | else
      |     fprintf('%s -- %s%s- %s Nexteer',NxtrConf,char(169),first,last)
      | end
  Out1 : Outport
  wires:
  In1/1 -> Out1/1

== system SF049A_LoaMgr/LoaMgr/LoaMgrPer1/Request_Responses/InvtrResp/Two/CopyRight2 ==

== system SF049A_LoaMgr/LoaMgr/LoaMgrPer1/Request_Responses/InvtrResp/Zero_or_Invalid/CopyRight2 ==

== system SF049A_LoaMgr/LoaMgr/LoaMgrPer1/Request_Responses/InvtrResp/one/CopyRight2 ==

== system SF049A_LoaMgr/LoaMgr/LoaMgrPer1/Request_Responses/MotAgResp/Three/CopyRight2 ==

== system SF049A_LoaMgr/LoaMgr/LoaMgrPer1/Request_Responses/MotAgResp/Two/CopyRight2 ==

== system SF049A_LoaMgr/LoaMgr/LoaMgrPer1/Request_Responses/MotAgResp/Zero_or_Invalid/CopyRight2 ==

== system SF049A_LoaMgr/LoaMgr/LoaMgrPer1/Request_Responses/MotAgResp/Zero_or_Invalid/cal1 ==
  In1 : Inport
  Action Port : ActionPort  ActionType=then
  CopyRight2 : Subsystem  Description=|  mask(Copyright Information){none=on}
      | Copyright info block.                                               
      |                                                                     
      | Place copyright information at the top of every subsystem in design.
      mask prompts: none "No parameters"
      mask help: Place copyright information at the top of every subsystem in design.
      mask Display:
      | NxtrConf = 'Nexteer Confidential';
      | 
      | sys = bdroot; %handle for the current model ("system")
      | first = get_param(sys,'Created');
      | first = first(end-3:end);  %year is last four digits
      | 
      | last = get_param(sys,'LastModifiedDate');
      | if isempty(last)
      |     last = datestr(now,'yyyy');
      | else
      |     last = last(end-3:end);
      | end
      | 
      | if strcmp(first,last)
      |     fprintf('%s -- Copyright %s Nexteer',NxtrConf,first)
      | else
      |     fprintf('%s -- %s%s- %s Nexteer',NxtrConf,char(169),first,last)
      | end
  Out2 : Outport
  wires:
  In1/1 -> Out2/1

== system SF049A_LoaMgr/LoaMgr/LoaMgrPer1/Request_Responses/MotAgResp/Zero_or_Invalid/cal2 ==
  In1 : Inport
  Action Port : ActionPort  ActionType=else
  CopyRight2 : Subsystem  Description=|  mask(Copyright Information){none=on}
      | Copyright info block.                                               
      |                                                                     
      | Place copyright information at the top of every subsystem in design.
      mask prompts: none "No parameters"
      mask help: Place copyright information at the top of every subsystem in design.
      mask Display:
      | NxtrConf = 'Nexteer Confidential';
      | 
      | sys = bdroot; %handle for the current model ("system")
      | first = get_param(sys,'Created');
      | first = first(end-3:end);  %year is last four digits
      | 
      | last = get_param(sys,'LastModifiedDate');
      | if isempty(last)
      |     last = datestr(now,'yyyy');
      | else
      |     last = last(end-3:end);
      | end
      | 
      | if strcmp(first,last)
      |     fprintf('%s -- Copyright %s Nexteer',NxtrConf,first)
      | else
      |     fprintf('%s -- %s%s- %s Nexteer',NxtrConf,char(169),first,last)
      | end
  Out1 : Outport
  wires:
  In1/1 -> Out1/1

== system SF049A_LoaMgr/LoaMgr/LoaMgrPer1/Request_Responses/MotAgResp/one/CopyRight2 ==
